simulink model "energy_storage"  (R2018a)
settings: Solver=ode4  StartTime=0.0  StopTime=simu.tTotal  FixedStep=simu.tStep  RelTol=1e-3
undefined symbols (not defined in the file or in its folder): D11, Delta, DiscIntNeverNeededParam, es1, es2, ess, flex, grid, gsc, gt1, ld, sim, simu, u0, Vbase, vsc, WT
libraries: powerlib x40, pwrsys x37, simulink x2, powerlib_meascontrol x2, simulink_extras x1, sps_avr x1
(part 1 of 2)
settings Model: SimulationMode=accelerator  Creator=ericfa  LastModifiedBy=ericfa
settings OptimizationCC: DefaultUnderspecifiedDataType=single
settings DebuggingCC: UnconnectedInputMsg=none  UnconnectedOutputMsg=none  UnconnectedLineMsg=none  UniqueDataStoreMsg=error  StrictBusMsg=ErrorOnBusTreatedAsVector

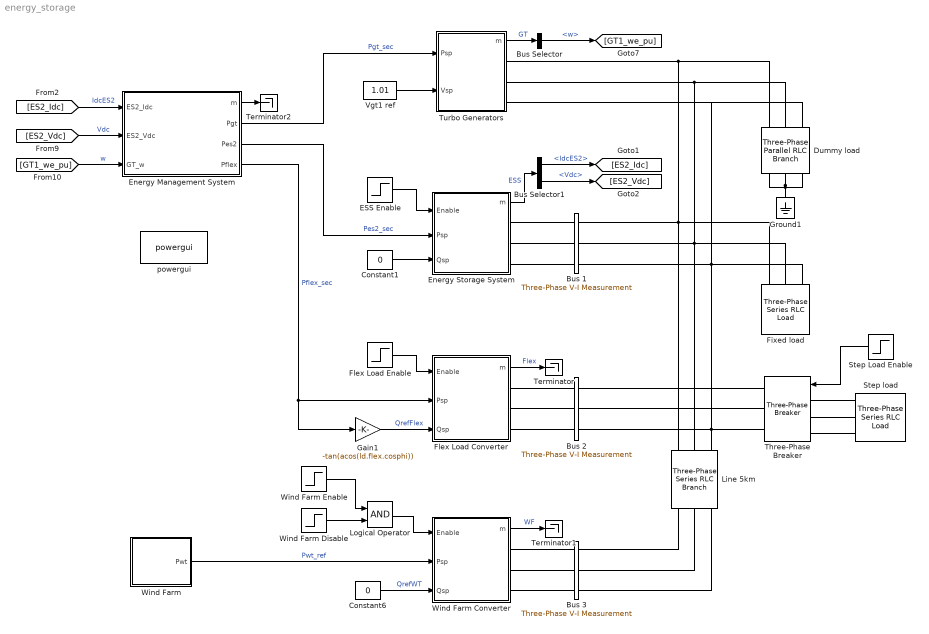
== system energy_storage ==
  Bus Selector : BusSelector  OutputSignals=w
  Bus Selector1 : BusSelector  OutputSignals=IdcES2,Vdc
  Bus 1 : powerlib/Measurements/Three-Phase V-I Measurement  VoltageMeasurement=no  SetLabelV=on  LabelV=Vabc_B2  Vpu=off  VpuLL=off  CurrentMeasurement=no  SetLabelI=on  LabelI=Iabc_B2  Ipu=off  Pbase=100e6  Vbase=500e3  OutputType=Magnitude  PhasorSimulation=off  PSBequivalent=0
      settings: SourceProductName=Simscape Electrical
  Bus 2 : powerlib/Measurements/Three-Phase V-I Measurement  VoltageMeasurement=no  SetLabelV=on  LabelV=Vabc_B2  Vpu=off  VpuLL=off  CurrentMeasurement=no  SetLabelI=on  LabelI=Iabc_B2  Ipu=off  Pbase=100e6  Vbase=500e3  OutputType=Magnitude  PhasorSimulation=off  PSBequivalent=0
      settings: SourceProductName=Simscape Electrical
  Bus 3 : powerlib/Measurements/Three-Phase V-I Measurement  VoltageMeasurement=no  SetLabelV=on  LabelV=Vabc_B2  Vpu=off  VpuLL=off  CurrentMeasurement=no  SetLabelI=on  LabelI=Iabc_B2  Ipu=off  Pbase=100e6  Vbase=500e3  OutputType=Magnitude  PhasorSimulation=off  PSBequivalent=0
      settings: SourceProductName=Simscape Electrical
  Constant1 : Constant  Value=0
  Constant6 : Constant  Value=0
  Dummy load : powerlib/Elements/Three-Phase Parallel RLC Branch  LConnTagsString=A|B|C  RConnTagsString=A|B|C  BranchType=R  Resistance=100*grid.UB2^2/grid.Sb  Inductance=1e-3  Capacitance=1e-6  Measurements=None
      settings: SourceProductName=Simscape Power Systems  SourceProductBaseCode=PS
  ESS Enable : Step  Time=4/grid.fn  SampleTime=0
  Energy Management System : Subsystem
  Energy Storage System : Subsystem
  Fixed load : powerlib/Elements/Three-Phase Series RLC Load  LConnTagsString=A|B|C  Configuration=Delta  NominalVoltage=grid.UB2  Vabc=[1e3 1e3 1e3]  Vabcp=[1e3 1e3 1e3]  NominalFrequency=grid.fn  UnbalancedPower=off  ActivePower=ld.fix.P  InductivePower=tan(acos(ld.fix.cosphi))*ld.fix.P  CapacitivePower=0  Pabc=[10e3 9e3 11e3]  QLabc=[100 90 110]  QCabc=[100 90 110]  Pabcp=[10e3 9e3 11e3]  QLabcp=[100 90 110]  QCabcp=[100 90 110]  Measurements=None  LoadType=constant Z
  Flex Load Converter : Subsystem
  Flex Load Enable : Step  Time=4/grid.fn  SampleTime=0
  Gain1 : Gain  Gain=-tan(acos(ld.flex.cosphi))
  Ground1 : powerlib/Elements/Ground  LConnTagsString=a
  Line 5km : powerlib/Elements/Three-Phase Series RLC Branch  LConnTagsString=A|B|C  RConnTagsString=A|B|C  BranchType=RL  Resistance=0.01273*5  Inductance=5*(0.2337e-3)  Capacitance=1e-6  Measurements=None
  Logical Operator : Logic  AllPortsSameDT=off  OutDataTypeStr=boolean
  Step Load Enable : Step  Time=simu.tLDstep  Before=ld.step.st  After=(1 - ld.step.st)  SampleTime=0
  Step load : powerlib/Elements/Three-Phase Series RLC Load  LConnTagsString=A|B|C  Configuration=Delta  NominalVoltage=grid.UB2  Vabc=[1e3 1e3 1e3]  Vabcp=[1e3 1e3 1e3]  NominalFrequency=grid.fn  UnbalancedPower=off  ActivePower=ld.step.P  InductivePower=tan(acos(ld.fix.cosphi))*ld.step.P  CapacitivePower=0  Pabc=[10e3 9e3 11e3]  QLabc=[100 90 110]  QCabc=[100 90 110]  Pabcp=[10e3 9e3 11e3]  QLabcp=[100 90 110]  QCabcp=[100 90 110]  Measurements=None  LoadType=constant Z
  Terminator : Terminator
  Terminator1 : Terminator
  Terminator2 : Terminator
  Three-Phase Breaker : powerlib/Elements/Three-Phase Breaker  InitialState=open  SwitchA=on  SwitchB=on  SwitchC=on  SwitchTimes="[1/60  5/60]"  External=on  BreakerResistance=0.01  SnubberResistance=1e6  SnubberCapacitance=inf  Measurements=None
  Turbo Generators : Subsystem  SystemSampleTime=10*sim.tStep  mask(Synchronous Generator with Exciter and Governor){SMVn=grid.UB2, SMPn=gt1.SM.Sn, SMcosphi=gt1.SM.cosphi, SMfn=grid.fn, SMp=gt1.SM.p, SMM=gt1.SM.M/2, SMXd=gt1.SM.Xd, SMXdp=gt1.SM.Xdp, SMXdpp=gt1.SM.Xdpp, SMXq=gt1.SM.Xq, SMXqpp=gt1.SM.Xqpp, SMXl=gt1.SM.Xl, SMRs=gt1.SM.Rs, SMTdpSC=gt1.SM.TdpSC, SMTdppSC=gt1.SM.TdppSC, SMTqppSC=gt1.SM.TqppSC, TurbT=gt1.Turb.T, GovKp=gt1.P.Kp, GovKd=gt1.P.Kd, GovTr=gt1.P.Tr, GovFlp=gt1.P.flp, GovDB=gt1.P.DB, ExcTr=gt1.exc.Tr, ExcKa=gt1.exc.Ka, ExcVRMax=gt1.exc.VRmax, ExcVRMin=gt1.exc.VRmin, ExcKf=gt1.exc.Kf, ExcTf=gt1.exc.Tf, ExcTb=gt1.exc.Tb, ExcTc=gt1.exc.Tc, ExcTb1=gt1.exc.Tb1, ExcTc1=gt1.exc.Tc1}
      mask prompts: SMVn "Voltage [V]"; SMPn "Apparent power [VA]"; SMcosphi "Power factor"; SMfn "Frequency [Hz]"; SMp "Pairs of poles"; SMM "Inertia constant [s]"; SMXd "d-axis steady-state"; SMXdp "d-axis transient"; SMXdpp "d-axis subtransient"; SMXq "q-axis steady-state"; SMXqpp "q-axis subtransient"; SMXl "Leakage"; SMRs "Stator (armature) resistance"; SMTdpSC "d-axis transient time"; SMTdppSC "d-axis subtransient time"; SMTqppSC "q-axis subtransient time"; TurbT "Equivalent first-order delay [s]"; GovKp "Permanent droop (primary control)"; GovKd "Transient droop (primary control)"; GovTr "Reset time transient droop (primary control)"; GovFlp "Low-pass frequency [Hz]"; GovDB "Deadband [pu]"; ExcTr "Input filter time constant [s]"; ExcKa "Proportional gain"; ExcVRMax "Maximum output [pu]"; ExcVRMin "Minimum output [pu]"; ExcKf "Rate feedback (derivative) gain"; ExcTf "Rate feedback (reset) time [s]"; ExcTb "1st lag time constant [s]"; ExcTc "1st lead time constant [s]"; ExcTb1 "2nd lag time constant [s]"; ExcTc1 "2nd lead time constant [s]"
      mask DialogControl ParameterGroupVar Prompt: Synchronous Machine
      mask DialogControl Container11_copy Prompt: Rated values
      mask DialogControl Container11 Prompt: Impedances [pu]
      mask DialogControl Container19 Prompt: Short-circuit time constants [s]
      mask DialogControl Container3 Prompt: Turbine
      mask DialogControl Container4 Prompt: Controllers
      mask DialogControl Container6 Prompt: Governor
      mask DialogControl Container8 Prompt: Exciter
  Vgt1 ref : Constant  Value=1.01
  Wind Farm : Subsystem
  Wind Farm Converter : Subsystem
  Wind Farm Disable : Step  Time=simu.tWToff  Before=1  After=0  SampleTime=0
  Wind Farm Enable : Step  Time=4/grid.fn  SampleTime=0
  powergui : powerlib/powergui  Priority=1  SimulationMode=Discrete  SampleTime=simu.tStep  frequency=60  Iterations=50  frequencyindice=0  Pbase=100e6  ErrMax=0.0001  UnitsV=kV  UnitsW=MW  buscounter=0  FunctionMessages=off  echomessages=off  EnableUseOfTLC=off  CurrentSourceSwitches=off  DisableSnubberDevices=off  DisableRonSwitches=off  DisableVfSwitches=off  DisplayEquations=off  SolverType=Tustin/Backward Euler (TBE)  Interpol=off  ExternalGateDelay=off  methode=off  Ts=100  x0status=blocks  SPID=on  SwTol=0  HookPort=off  RestoreLinks=warning  ResistiveCurrentMeasurement=off  Frange=[0:2:500]  Ylog=off  Xlog=on  ShowGrid=off  save=off  variable=ZData  structure=0  ZoomFFT=off  StartTime=0.0  cycles=1  DisplayStyle=1  fundamental=60  FreqAxis=off  MaxFrequency=1000  frequencyindicesteady=1  RmsSteady=2  display=off
  wires:
  ESS Enable/1 -> Energy Storage System/1(Enable)
  Constant1/1 -> Energy Storage System/3(Qsp)
  Vgt1 ref/1 -> Turbo Generators/2(Vsp)
  Gain1/1 -> Flex Load Converter/3(Qsp)  "QrefFlex"
  Flex Load Enable/1 -> Flex Load Converter/1(Enable)
  Energy Management System/4(Pflex) -> Gain1/1, Flex Load Converter/2(Psp)  "Pflex_sec"
  Constant6/1 -> Wind Farm Converter/3(Qsp)  "QrefWT"
  Wind Farm Enable/1 -> Logical Operator/1
  Wind Farm/1(Pwt) -> Wind Farm Converter/2(Psp)  "Pwt_ref"
  Step Load Enable/1 -> Three-Phase Breaker/1
  Bus Selector/1 -> [GT1_we_pu]  "<w>"
  Turbo Generators/1(m) -> Bus Selector/1  "GT"
  Flex Load Converter/1(m) -> Terminator/1  "Flex"
  Wind Farm Converter/1(m) -> Terminator1/1  "WF"
  Bus Selector1/1 -> [ES2_Idc]  "<IdcES2>"
  Energy Storage System/1(m) -> Bus Selector1/1  "ESS"
  Bus Selector1/2 -> [ES2_Vdc]  "<Vdc>"
  [ES2_Idc] -> Energy Management System/1(ES2_Idc)  "IdcES2"
  [ES2_Vdc] -> Energy Management System/2(ES2_Vdc)  "Vdc"
  [GT1_we_pu] -> Energy Management System/3(GT_w)  "w"
  Energy Management System/2(Pgt) -> Turbo Generators/1(Psp)  "Pgt_sec"
  Energy Management System/3(Pes2) -> Energy Storage System/2(Psp)  "Pes2_sec"
  Energy Management System/1(m) -> Terminator2/1
  Wind Farm Disable/1 -> Logical Operator/2
  Logical Operator/1 -> Wind Farm Converter/1(Enable)
  connections:
  Dummy load/LConn2 -- Turbo Generators/RConn2 -- Fixed load/LConn2 -- Three-Phase Breaker/RConn2 -- Line 5km/LConn2 -- Bus 2/RConn2 -- Bus 1/RConn2
  Three-Phase Breaker/RConn3 -- Dummy load/LConn3 -- Turbo Generators/RConn3 -- Fixed load/LConn3 -- Bus 1/RConn3 -- Line 5km/LConn3 -- Bus 2/RConn3
  Energy Storage System/RConn1 -- Bus 1/LConn1
  Energy Storage System/RConn2 -- Bus 1/LConn2
  Energy Storage System/RConn3 -- Bus 1/LConn3
  Dummy load/LConn1 -- Turbo Generators/RConn1 -- Fixed load/LConn1 -- Three-Phase Breaker/RConn1 -- Line 5km/LConn1 -- Bus 2/RConn1 -- Bus 1/RConn1
  Dummy load/RConn2 -- Dummy load/RConn3 -- Dummy load/RConn1 -- Ground1/LConn1
  Flex Load Converter/RConn1 -- Bus 2/LConn1
  Flex Load Converter/RConn2 -- Bus 2/LConn2
  Flex Load Converter/RConn3 -- Bus 2/LConn3
  Wind Farm Converter/RConn3 -- Bus 3/LConn3
  Wind Farm Converter/RConn2 -- Bus 3/LConn2
  Wind Farm Converter/RConn1 -- Bus 3/LConn1
  Bus 3/RConn1 -- Line 5km/RConn1
  Bus 3/RConn2 -- Line 5km/RConn2
  Bus 3/RConn3 -- Line 5km/RConn3
  Step load/LConn1 -- Three-Phase Breaker/LConn1
  Step load/LConn2 -- Three-Phase Breaker/LConn2
  Step load/LConn3 -- Three-Phase Breaker/LConn3

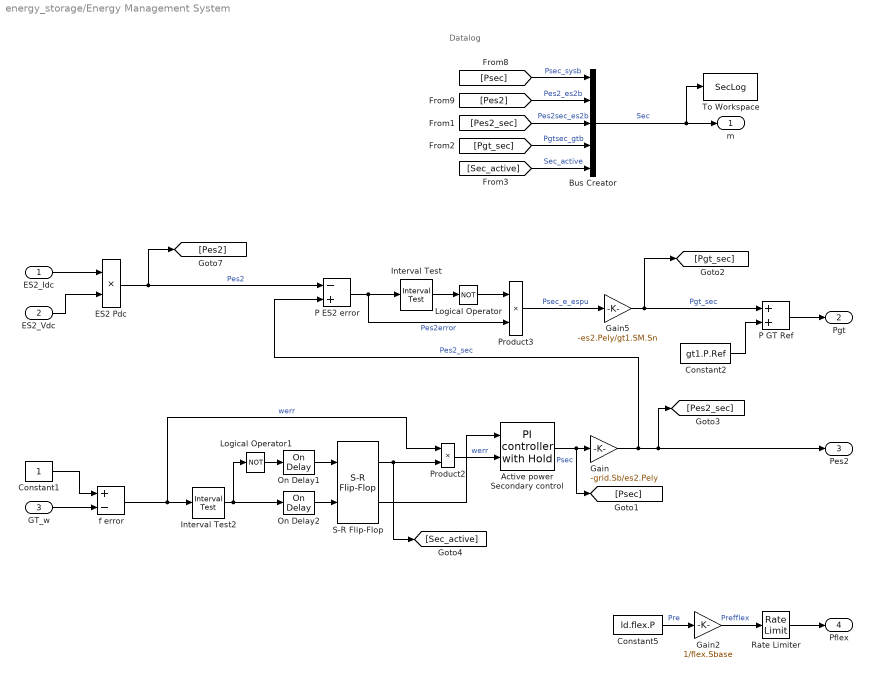
== system energy_storage/Energy Management System ==
  note: Datalog
  ES2_Idc : Inport
  ES2_Vdc : Inport  Port=2
  GT_w : Inport  Port=3
  Active power Secondary control : pwrsys/Controllers/PI controller  with Hold  Kp=0.05  Ki=gt1.P.Ki  Max=(es2.Pfc + gt1.SM.Sn*gt1.SM.cosphi-gt1.P.Ref*gt1.SM.Sn)/grid.Sb  Min=-(es2.Pely+gt1.P.Ref*gt1.SM.Sn)/grid.Sb  x0=0  Ts=10/grid.fn
      settings: SourceProductName=NTNU Power Systems
  Bus Creator : BusCreator  Inputs=5
  Constant1 : Constant
  Constant2 : Constant  Value=gt1.P.Ref
  Constant5 : Constant  Value=ld.flex.P
  ES2 Pdc : Product
  Gain : Gain  Gain=-grid.Sb/es2.Pely
  Gain2 : Gain  Gain=1/flex.Sbase
  Gain5 : Gain  Gain=-es2.Pely/gt1.SM.Sn
  Interval Test : simulink/Logic and Bit Operations/Interval Test  IntervalClosedRight=on  uplimit=0.05  IntervalClosedLeft=on  lowlimit=-0.05  OutDataTypeStr=boolean
  Interval Test2 : simulink/Logic and Bit Operations/Interval Test  IntervalClosedRight=on  uplimit=0.005  IntervalClosedLeft=on  lowlimit=-0.005  OutDataTypeStr=boolean
  Logical Operator : Logic  Operator=NOT  AllPortsSameDT=off  OutDataTypeStr=boolean
  Logical Operator1 : Logic  Operator=NOT  AllPortsSameDT=off  OutDataTypeStr=boolean
  On Delay1 : powerlib_meascontrol/Logic/On Delay  DelayType=On delay  delay=30  ic=0  Ts=10/grid.fn
      settings: SourceProductName=Simscape Power Systems
  On Delay2 : powerlib_meascontrol/Logic/On Delay  DelayType=On delay  delay=60  ic=0  Ts=10/grid.fn
      settings: SourceProductName=Simscape Power Systems
  P ES2 error : Sum  Inputs=-+
  P GT Ref : Sum
  Product2 : Product
  Product3 : Product
  Rate Limiter : RateLimiter  RisingSlewLimit=100  FallingSlewLimit=-100  SampleTimeMode=inherited
  S-R Flip-Flop : simulink_extras/Flip Flops/S-R Flip-Flop  initial_condition=0
  To Workspace : ToWorkspace  VariableName=SecLog  SaveFormat=Timeseries  SampleTime=-1
      settings: Decimation=2000
  f error : Sum  Inputs=+-
  m : Outport
  Pgt : Outport  Port=2
  Pes2 : Outport  Port=3
  Pflex : Outport  Port=4
  wires:
  Constant1/1 -> f error/1
  Product2/1 -> Active power Secondary control/2  "werr"
  Product3/1 -> Gain5/1  "Psec_e_espu"
  Gain/1 -> [Pes2_sec], Pes2/1, P ES2 error/2  "Pes2_sec"
  P ES2 error/1 -> Interval Test/1, Product3/2  "Pes2error"
  Active power Secondary control/1 -> [Psec], Gain/1  "Psec"
  Interval Test2/1 -> Logical Operator1/1, On Delay2/1
  S-R Flip-Flop/2 -> Active power Secondary control/1
  GT_w/1 -> f error/2
  On Delay2/1 -> S-R Flip-Flop/2
  Logical Operator1/1 -> On Delay1/1
  f error/1 -> Product2/1, Interval Test2/1  "werr"
  S-R Flip-Flop/1 -> [Sec_active], Product2/2
  Interval Test/1 -> Logical Operator/1
  Logical Operator/1 -> Product3/1
  On Delay1/1 -> S-R Flip-Flop/1
  ES2 Pdc/1 -> [Pes2], P ES2 error/1  "Pes2"
  ES2_Idc/1 -> ES2 Pdc/1
  ES2_Vdc/1 -> ES2 Pdc/2
  Gain5/1 -> P GT Ref/1, [Pgt_sec]  "Pgt_sec"
  Bus Creator/1 -> To Workspace/1, m/1  "Sec"
  [Pes2_sec] -> Bus Creator/3  "Pes2sec_es2b"
  [Pgt_sec] -> Bus Creator/4  "Pgtsec_gtb"
  [Psec] -> Bus Creator/1  "Psec_sysb"
  [Pes2] -> Bus Creator/2  "Pes2_es2b"
  [Sec_active] -> Bus Creator/5  "Sec_active"
  Constant5/1 -> Gain2/1  "Pre"
  Gain2/1 -> Rate Limiter/1  "Prefflex"
  Rate Limiter/1 -> Pflex/1
  Constant2/1 -> P GT Ref/2
  P GT Ref/1 -> Pgt/1

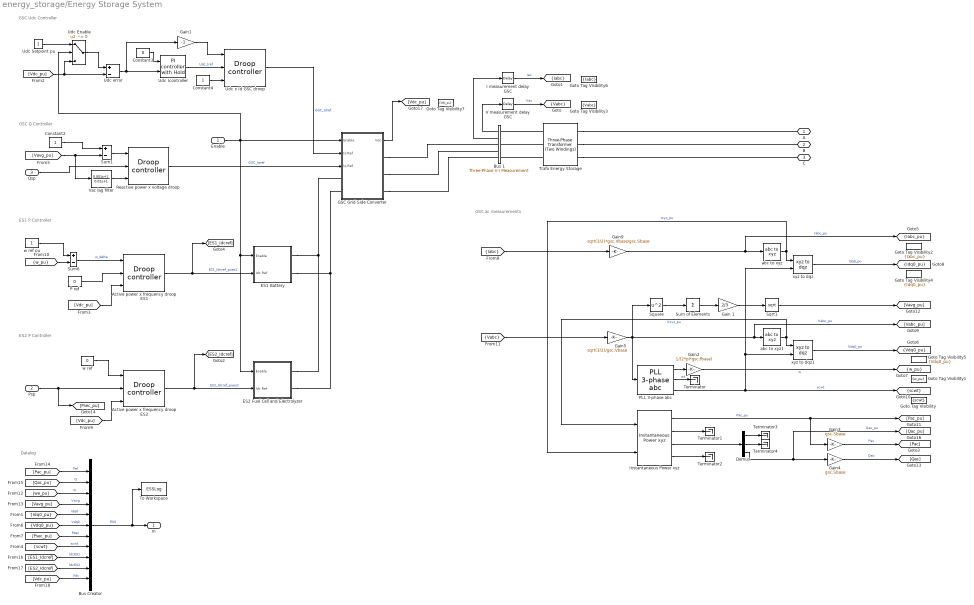
== system energy_storage/Energy Storage System ==
  note: GSC ac measurements
  note: ES1 P Controller
  note: GSC Q Controller
  note: GSC Udc Controller
  note: ES2 P Controller
  note: Datalog
  Enable : Inport
  Psp : Inport  Port=2
  Qsp : Inport  Port=3
  Active power x frequency droop ES1 : pwrsys/Controllers/Droop controller  Refmax=1  Refmin=-1  Ts=-1  Kp=ess.P.Kp  Kd=0  Tr=ess.P.Tr  flp=ess.P.flp  DB=ess.P.DB
      settings: SourceProductName=NTNU Power Systems
  Active power x frequency droop ES2 : pwrsys/Controllers/Droop controller  Refmax=1  Refmin=-es2.Pfc/es2.Pely  Ts=-1  Kp=0  Kd=0  Tr=ess.P.Tr  flp=ess.P.flp  DB=ess.P.DB
      settings: SourceProductName=NTNU Power Systems
  Bus Creator : BusCreator  Inputs=11
  Bus 1 : powerlib/Measurements/Three-Phase V-I Measurement  VoltageMeasurement=phase-to-ground  SetLabelV=off  LabelV=Vabc  Vpu=off  VpuLL=off  CurrentMeasurement=yes  SetLabelI=off  LabelI=Iabc  Ipu=off  Pbase=Sbase  Vbase=Vbase*sqrt(3/2)  OutputType=Complex  PhasorSimulation=off  PSBequivalent=0
  Constant2 : Constant
  Constant3 : Constant  Value=0
  Constant4 : Constant
  Demux : Demux  Outputs=3
  ES1 Battery : Subsystem
  ES2 Fuel Cell and Electrolyzer : Subsystem
  GSC Grid Side Converter : Subsystem
  "Gain 1 " : Gain  Gain=2/3
  Gain1 : Gain  Gain=-1
  Gain2 : Gain  Gain=1/(2*pi*gsc.fbase)
  Gain3 : Gain  Gain=gsc.Sbase
  Gain4 : Gain  Gain=gsc.Sbase
  Gain5 : Gain  Gain=sqrt(3/2)/gsc.Vbase
  Gain9 : Gain  Gain=sqrt(3/2)*gsc.Vbase/gsc.Sbase
  Goto Tag Visibility : GotoTagVisibility  GotoTag=scwt
  Goto Tag Visibility1 : GotoTagVisibility  GotoTag=w_pu
  Goto Tag Visibility2 : GotoTagVisibility  GotoTag=Iabc_pu
  Goto Tag Visibility3 : GotoTagVisibility  GotoTag=Vabc
  Goto Tag Visibility4 : GotoTagVisibility  GotoTag=Idq0_pu
  Goto Tag Visibility5 : GotoTagVisibility  GotoTag=Vdq0_pu
  Goto Tag Visibility6 : GotoTagVisibility  GotoTag=Iabc
  Goto Tag Visibility7 : GotoTagVisibility  GotoTag=Vdc_pu
  I measurement delay GSC : TransportDelay  DelayTime=simu.tStep
  Instantaneous Power xyz : pwrsys/Measurement/Instantaneous Power xyz  typeTransf=Amplitude-invariant
      settings: SourceProductName=NTNU Power Systems
  P ref : Constant  Value=0
  PLL 3-phase abc : pwrsys/PLLs/PLL 3-phase abc  fnom=gsc.fbase  fdev=1/3*gsc.fbase  zeta=0.707  Kp=gsc.pll.Kp  Ki=gsc.pll.Ki  Kd=gsc.pll.Kd  Tr=gsc.pll.Tr  Ts=gsc.fSwitch  wt0=0
      settings: SourceProductName=NTNU Power Systems
  Reactive power x voltage droop : pwrsys/Controllers/Droop controller  Refmax=1  Refmin=-1  Ts=-1  Kp=ess.Q.Kp  Kd=ess.Q.Kd  Tr=ess.Q.Tr  flp=ess.Q.flp  DB=ess.Q.DB
      settings: SourceProductName=NTNU Power Systems
  Sqrt1 : Sqrt  SaturateOnIntegerOverflow=on
  Square : Math  Operator=square  SaturateOnIntegerOverflow=on
  Sum of Elements : Sum  Inputs=+
  Sum1 : Sum  Inputs=+-
  Sum6 : Sum  Inputs=+-
  Terminator{,1..4} (5 alike) : Terminator
  To Workspace : ToWorkspace  VariableName=ESSLog  SaveFormat=Timeseries  SampleTime=-1
      settings: Decimation=20
  Trafo Energy Storage : powerlib/Elements/Three-Phase Transformer (Two Windings)  Winding1Connection=Yg  Winding2Connection=Delta (D11)  CoreType=Three single-phase transformers  SetSaturation=off  Hysteresis=off  DataFile='hysteresis'  SetInitialFlux=off  Measurements=None  UNITS=pu  NominalPower=[ gsc.Sbase , grid.fn ]  Winding1=[ grid.UB1 , 0.002 , gsc.filterpu.Lg/2 ]  Winding2=[ grid.UB2 , 0.002 , gsc.filterpu.Lg/2 ]  Rm=200  Lm=200  L0=0.5  Saturation=[ 0,0 ; 0.0024,1.2 ; 1.0,1.52 ]  InitialFluxes=[ 0.8 , -0.8 , 0.7 ]  MoreParameters=off  BreakLoop=off  DataType=off  TransfoNumber=1
  Udc Enable : Switch  Criteria=u2 ~= 0
  Udc Icontroller : pwrsys/Controllers/PI controller  with Hold  Kp=0  Ki=ess.Udc.Ki  Max=1  Min=-1  x0=0  Ts=-1
      settings: SourceProductName=NTNU Power Systems
  Udc Setpoint pu : Constant
  Udc error : Sum  Inputs=+-
  "Udc x Id GSC droop " : pwrsys/Controllers/Droop controller  Refmax=1  Refmin=-1  Ts=-1  Kp=ess.Udc.Kp  Kd=ess.Udc.Kd  Tr=ess.Udc.Tr  flp=ess.Udc.flp  DB=ess.Udc.DB
      settings: SourceProductName=NTNU Power Systems
  V measurement delay GSC : TransportDelay  DelayTime=simu.tStep
  Vac lag filter : TransferFcn  Numerator=[0.001 1]  Denominator=[0.01 1]
  abc to xyz : pwrsys/Transformations/abc to xyz  typeTransf=Amplitude-invariant
      settings: SourceProductName=NTNU Power Systems
  abc to xyz1 : pwrsys/Transformations/abc to xyz  typeTransf=Amplitude-invariant
      settings: SourceProductName=NTNU Power Systems
  "w ref " : Constant  Value=0
  w ref pu : Constant
  xyz to dqz : pwrsys/Transformations/xyz to dqz  SystemSampleTime=-1
      settings: SourceProductName=NTNU Power Systems
  xyz to dqz1 : pwrsys/Transformations/xyz to dqz  SystemSampleTime=-1
      settings: SourceProductName=NTNU Power Systems
  A : PMIOPort  Side=Right
  B : PMIOPort  Port=2  Side=Right
  C : PMIOPort  Port=3  Side=Right
  m : Outport
  tag scope: Iabc=scoped, Iabc_pu=scoped, Idq0_pu=scoped, Vabc=scoped, Vdq0_pu=scoped, scwt=scoped, w_pu=scoped
  wires:
  Constant3/1 -> Udc Icontroller/1
  Udc Enable/1 -> Udc error/1
  Udc Setpoint pu/1 -> Udc Enable/1
  Udc error/1 -> Gain1/1, Udc Icontroller/2
  "Udc x Id GSC droop "/1 -> GSC Grid Side Converter/2(Id Ref)  "GSC_Idref"
  I measurement delay GSC/1 -> [Iabc]  "Iac"
  Active power x frequency droop ES1/1 -> ES1 Battery/2(Idc Ref), [ES1_Idcref]  "ES1_Idcref_pues1"
  [Vdc_pu] -> Udc Enable/3, Udc error/2
  V measurement delay GSC/1 -> [Vabc]  "Vac"
  Bus 1/1 -> V measurement delay GSC/1
  Udc Icontroller/1 -> "Udc x Id GSC droop "/2  "Udc_Iref"
  Constant2/1 -> Sum1/1
  w ref pu/1 -> Sum6/1
  Sum1/1 -> Reactive power x voltage droop/1
  Gain1/1 -> "Udc x Id GSC droop "/1
  Bus 1/2 -> I measurement delay GSC/1
  [w_pu] -> Sum6/2
  Sum6/1 -> Active power x frequency droop ES1/1  "w_delta"
  [Vdc_pu] -> Active power x frequency droop ES1/3
  Enable/1 -> ES2 Fuel Cell and Electrolyzer/1(Enable), ES1 Battery/1(Enable), GSC Grid Side Converter/1(Enable), Udc Enable/2
  Constant4/1 -> "Udc x Id GSC droop "/3
  Reactive power x voltage droop/1 -> GSC Grid Side Converter/3(Iq Ref)  "GSC_Iqref"
  [Vdc_pu] -> Active power x frequency droop ES2/3
  Active power x frequency droop ES2/1 -> ES2 Fuel Cell and Electrolyzer/2(Idc Ref), [ES2_Idcref]  "ES2_Idcref_pues2"
  "w ref "/1 -> Active power x frequency droop ES2/1
  P ref/1 -> Active power x frequency droop ES1/2
  [Vavg_pu] -> Vac lag filter/1, Sum1/2
  Vac lag filter/1 -> Reactive power x voltage droop/3
  Psp/1 -> [Psec_pu], Active power x frequency droop ES2/2
  Qsp/1 -> Reactive power x voltage droop/2
  Sqrt1/1 -> [Vavg_pu]
  Gain9/1 -> [Iabc_pu], abc to xyz/1  "Iabc_pu"
  xyz to dqz/1 -> [Idq0_pu]  "Idq0_pu"
  Gain5/1 -> Square/1, PLL 3-phase abc/1, [Vabc_pu], abc to xyz1/1  "Vabc_pu"
  PLL 3-phase abc/3 -> [scwt], xyz to dqz/2, xyz to dqz1/2  "scwt"
  Gain2/1 -> [w_pu]  "w"
  PLL 3-phase abc/1 -> Gain2/1
  xyz to dqz1/1 -> [Vdq0_pu]  "Vdq0_pu"
  [Iabc] -> Gain9/1
  [Vabc] -> Gain5/1
  Instantaneous Power xyz/1 -> Gain3/1, [Pac_pu]  "Pac_pu"
  Demux/3 -> [Qac_pu], Gain4/1  "Qac_pu"
  Square/1 -> Sum of Elements/1
  Sum of Elements/1 -> "Gain 1 "/1
  "Gain 1 "/1 -> Sqrt1/1
  abc to xyz/1 -> xyz to dqz/1, Instantaneous Power xyz/2  "Ixyz_pu"
  abc to xyz1/1 -> xyz to dqz1/1, Instantaneous Power xyz/1  "Vxyz_pu"
  PLL 3-phase abc/2 -> Terminator/1  "wt"
  Instantaneous Power xyz/2 -> Terminator1/1
  Instantaneous Power xyz/4 -> Terminator2/1
  Instantaneous Power xyz/3 -> Demux/1
  Demux/1 -> Terminator3/1
  Demux/2 -> Terminator4/1
  Gain3/1 -> [Pac]  "Pac"
  Gain4/1 -> [Qac]  "Qac"
  GSC Grid Side Converter/1(Vdc) -> [Vdc_pu]
  Bus Creator/1 -> To Workspace/1, m/1  "ESS"
  [Vavg_pu] -> Bus Creator/4  "Vavg"
  [Pac_pu] -> Bus Creator/1  "Pel"
  [Psec_pu] -> Bus Creator/7  "Psec"
  [Vdq0_pu] -> Bus Creator/6  "Vdq0"
  [Idq0_pu] -> Bus Creator/5  "Idq0"
  [Qac_pu] -> Bus Creator/2  "Q"
  [scwt] -> Bus Creator/8  "scwt"
  [we_pu] -> Bus Creator/3  "w"
  [ES1_Idcref] -> Bus Creator/9  "IdcES1"
  [ES2_Idcref] -> Bus Creator/10  "IdcES2"
  [Vdc_pu] -> Bus Creator/11  "Vdc"
  connections:
  ES1 Battery/RConn2 -- ES2 Fuel Cell and Electrolyzer/RConn2 -- GSC Grid Side Converter/LConn2
  Trafo Energy Storage/LConn2 -- Bus 1/LConn2
  GSC Grid Side Converter/RConn3 -- Bus 1/RConn3
  GSC Grid Side Converter/RConn1 -- Bus 1/RConn1
  Trafo Energy Storage/LConn3 -- Bus 1/LConn3
  GSC Grid Side Converter/RConn2 -- Bus 1/RConn2
  Trafo Energy Storage/LConn1 -- Bus 1/LConn1
  Trafo Energy Storage/RConn3 -- C/RConn1
  Trafo Energy Storage/RConn2 -- B/RConn1
  Trafo Energy Storage/RConn1 -- A/RConn1
  ES1 Battery/RConn1 -- ES2 Fuel Cell and Electrolyzer/RConn1 -- GSC Grid Side Converter/LConn1

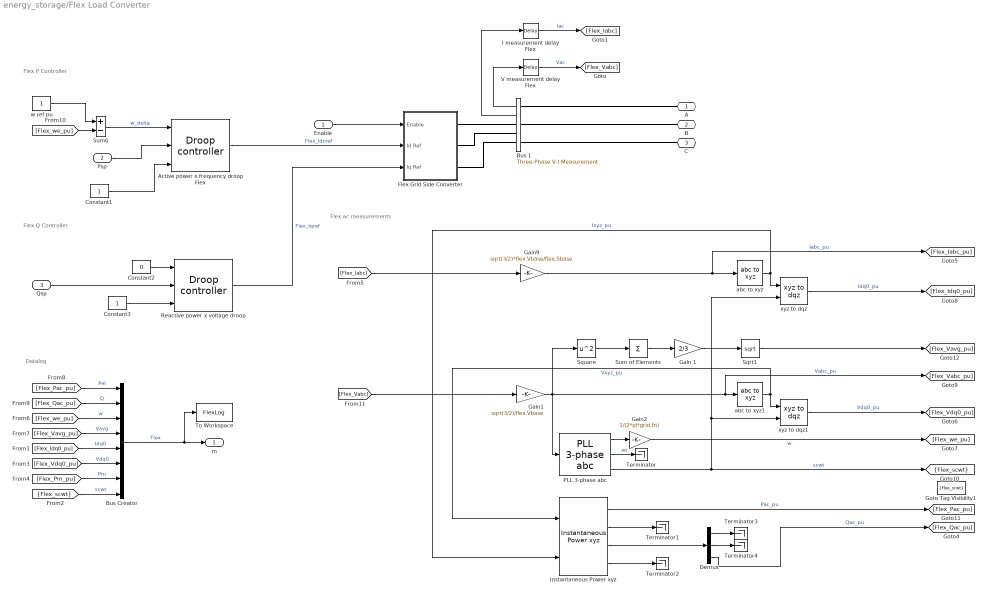
== system energy_storage/Flex Load Converter ==
  note: Flex ac measurements
  note: Flex P Controller
  note: Flex Q Controller
  note: Datalog
  Enable : Inport
  Psp : Inport  Port=2
  Qsp : Inport  Port=3
  Active power x frequency droop Flex : pwrsys/Controllers/Droop controller  Refmax=1  Refmin=0  Ts=-1  Kp=flex.P.Kp  Kd=0  Tr=flex.P.Tr  flp=flex.P.flp  DB=flex.P.DB
      settings: SourceProductName=NTNU Power Systems
  Bus Creator : BusCreator  Inputs=8
  Bus 1 : powerlib/Measurements/Three-Phase V-I Measurement  VoltageMeasurement=phase-to-ground  SetLabelV=off  LabelV=Vabc  Vpu=off  VpuLL=off  CurrentMeasurement=yes  SetLabelI=off  LabelI=Iabc  Ipu=off  Pbase=Sbase  Vbase=Vbase*sqrt(3/2)  OutputType=Complex  PhasorSimulation=off  PSBequivalent=0
  Constant1 : Constant
  Constant2 : Constant  Value=0
  Constant3 : Constant
  Demux : Demux  Outputs=3
  Flex Grid Side Converter : Subsystem
  "Gain 1 " : Gain  Gain=2/3
  Gain1 : Gain  Gain=sqrt(3/2)/flex.Vbase
  Gain2 : Gain  Gain=1/(2*pi*grid.fn)
  Gain9 : Gain  Gain=sqrt(3/2)*flex.Vbase/flex.Sbase
  Goto Tag Visibility1 : GotoTagVisibility  GotoTag=Flex_scwt
  I measurement delay Flex : TransportDelay  DelayTime=simu.tStep
  Instantaneous Power xyz : pwrsys/Measurement/Instantaneous Power xyz  typeTransf=Amplitude-invariant
      settings: SourceProductName=NTNU Power Systems
  PLL 3-phase abc : pwrsys/PLLs/PLL 3-phase abc  fnom=gsc.fbase  fdev=1/3*gsc.fbase  zeta=0.707  Kp=gsc.pll.Kp  Ki=gsc.pll.Ki  Kd=gsc.pll.Kd  Tr=gsc.pll.Tr  Ts=gsc.fSwitch  wt0=0
      settings: SourceProductName=NTNU Power Systems
  Reactive power x voltage droop : pwrsys/Controllers/Droop controller  Refmax=0.5  Refmin=-0.5  Ts=-1  Kp=0  Kd=0  Tr=1  flp=1  DB=0
      settings: SourceProductName=NTNU Power Systems
  Sqrt1 : Sqrt  SaturateOnIntegerOverflow=on
  Square : Math  Operator=square  SaturateOnIntegerOverflow=on
  Sum of Elements : Sum  Inputs=+
  Sum6 : Sum  Inputs=+-
  Terminator{,1..4} (5 alike) : Terminator
  To Workspace : ToWorkspace  VariableName=FlexLog  SaveFormat=Timeseries  SampleTime=-1
      settings: Decimation=20
  V measurement delay Flex : TransportDelay  DelayTime=simu.tStep
  abc to xyz : pwrsys/Transformations/abc to xyz  typeTransf=Amplitude-invariant
      settings: SourceProductName=NTNU Power Systems
  abc to xyz1 : pwrsys/Transformations/abc to xyz  typeTransf=Amplitude-invariant
      settings: SourceProductName=NTNU Power Systems
  w ref pu : Constant
  xyz to dqz : pwrsys/Transformations/xyz to dqz  SystemSampleTime=-1
      settings: SourceProductName=NTNU Power Systems
  xyz to dqz1 : pwrsys/Transformations/xyz to dqz  SystemSampleTime=-1
      settings: SourceProductName=NTNU Power Systems
  A : PMIOPort  Side=Right
  B : PMIOPort  Port=2  Side=Right
  C : PMIOPort  Port=3  Side=Right
  m : Outport
  tag scope: Flex_scwt=scoped
  wires:
  I measurement delay Flex/1 -> [Flex_Iabc]  "Iac"
  Active power x frequency droop Flex/1 -> Flex Grid Side Converter/2(Id Ref)  "Flex_Idcref"
  Enable/1 -> Flex Grid Side Converter/1(Enable)
  V measurement delay Flex/1 -> [Flex_Vabc]  "Vac"
  Bus 1/1 -> V measurement delay Flex/1
  Constant3/1 -> Reactive power x voltage droop/3
  w ref pu/1 -> Sum6/1
  Constant2/1 -> Reactive power x voltage droop/1
  Qsp/1 -> Reactive power x voltage droop/2
  Bus 1/2 -> I measurement delay Flex/1
  [Flex_we_pu] -> Sum6/2
  Sum6/1 -> Active power x frequency droop Flex/1  "w_delta"
  Constant1/1 -> Active power x frequency droop Flex/3
  Reactive power x voltage droop/1 -> Flex Grid Side Converter/3(Iq Ref)  "Flex_Iqref"
  Psp/1 -> Active power x frequency droop Flex/2
  [Flex_scwt] -> Bus Creator/8  "scwt"
  [Flex_we_pu] -> Bus Creator/3  "w"
  [Flex_Vdq0_pu] -> Bus Creator/6  "Vdq0"
  [Flex_Idq0_pu] -> Bus Creator/5  "Idq0"
  [Flex_Qac_pu] -> Bus Creator/2  "Q"
  [Flex_Pm_pu] -> Bus Creator/7  "Pm"
  [Flex_Vavg_pu] -> Bus Creator/4  "Vavg"
  Bus Creator/1 -> To Workspace/1, m/1  "Flex"
  [Flex_Pac_pu] -> Bus Creator/1  "Pel"
  Sqrt1/1 -> [Flex_Vavg_pu]
  Gain9/1 -> [Flex_Iabc_pu], abc to xyz/1  "Iabc_pu"
  xyz to dqz/1 -> [Flex_Idq0_pu]  "Idq0_pu"
  Gain1/1 -> Square/1, PLL 3-phase abc/1, [Flex_Vabc_pu], abc to xyz1/1  "Vabc_pu"
  PLL 3-phase abc/3 -> [Flex_scwt], xyz to dqz/2, xyz to dqz1/2  "scwt"
  Gain2/1 -> [Flex_we_pu]  "w"
  PLL 3-phase abc/1 -> Gain2/1
  xyz to dqz1/1 -> [Flex_Vdq0_pu]  "Vdq0_pu"
  [Flex_Iabc] -> Gain9/1
  [Flex_Vabc] -> Gain1/1
  Instantaneous Power xyz/1 -> [Flex_Pac_pu]  "Pac_pu"
  Demux/3 -> [Flex_Qac_pu]  "Qac_pu"
  Square/1 -> Sum of Elements/1
  Sum of Elements/1 -> "Gain 1 "/1
  "Gain 1 "/1 -> Sqrt1/1
  abc to xyz/1 -> xyz to dqz/1, Instantaneous Power xyz/2  "Ixyz_pu"
  abc to xyz1/1 -> xyz to dqz1/1, Instantaneous Power xyz/1  "Vxyz_pu"
  PLL 3-phase abc/2 -> Terminator/1  "wt"
  Instantaneous Power xyz/2 -> Terminator1/1
  Instantaneous Power xyz/4 -> Terminator2/1
  Instantaneous Power xyz/3 -> Demux/1
  Demux/1 -> Terminator3/1
  Demux/2 -> Terminator4/1
  connections:
  B/RConn1 -- Bus 1/LConn2
  Bus 1/RConn3 -- Flex Grid Side Converter/RConn3
  Bus 1/RConn1 -- Flex Grid Side Converter/RConn1
  C/RConn1 -- Bus 1/LConn3
  Bus 1/RConn2 -- Flex Grid Side Converter/RConn2
  A/RConn1 -- Bus 1/LConn1

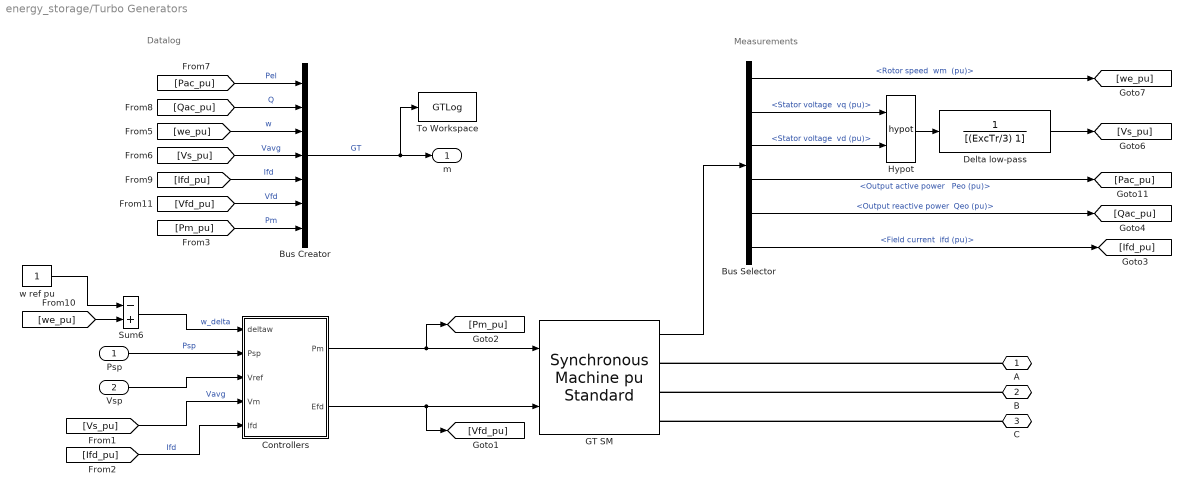
== system energy_storage/Turbo Generators ==
  note: Measurements
  note: Datalog
  Psp : Inport
  Vsp : Inport  Port=2
  Bus Creator : BusCreator  Inputs=7
  Bus Selector : BusSelector  OutputSignals="Mechanical.Rotor speed  wm  (pu),dq0 components.Stator voltage  vq (pu),dq0 components.Stator voltage  vd (pu),Output active power   Peo (pu),Output reactive power  Qeo (pu),dq0 components.Field current  ifd (pu)"
  Controllers : Subsystem  SystemSampleTime=1/(20*grid.fn)
  Delta low-pass : TransferFcn  Denominator=[(ExcTr/3) 1]
  GT SM : powerlib/Machines/Synchronous Machine pu Standard  PresetModel=No  MechanicalLoad=Mechanical power Pm  ShowDetailedParameters=on  RotorType=Salient-pole  Units=per unit standard parameters  MeasurementBus=off  NominalParameters=[SMPn SMVn SMfn]  Reactances1=[ 2.12, 0.299, 0.188, 1.76, 0.65, 0.25, 0.15 ]  Reactances2=[SMXd SMXdp SMXdpp SMXq SMXqpp SMXl]  dAxisTimeConstants=Short-circuit  qAxisTimeConstants=Short-circuit  TimeConstants1="[ 4.4849  0.0681  0.1  ]"  TimeConstants2=[ 8.0, 0.03, 1.0, 0.07 ]  TimeConstants3="[  4.49  0.0681  0.0513  ]"  TimeConstants4=[ 8.0, 0.03, 0.3371, 0.0295 ]  TimeConstants5=[ 1.01, 0.053, 0.1 ]  TimeConstants6=[ 1.3201, 0.023, 1.0, 0.07 ]  TimeConstants7=[SMTdpSC SMTdppSC SMTqppSC]  TimeConstants8=[ 1.3201, 0.0231, 0.3371, 0.0295 ]  StatorResistance=SMRs  Mechanical=[SMM 0 SMp]  PolePairs=20  InitialConditions=[0 -67.7688 0.420455 0.420455 0.420455 0 -120 120 sqrt(3/2)*1.27233]  SetSaturation=on  Saturation=[0.6404,0.7127,0.8441,0.9214,0.9956,1.082,1.19,1.316,1.457;0.7,0.7698,0.8872,0.9466,0.9969,1.046,1.1,1.151,1.201]  LoadFlowParameters=[2 37000000 0 0 0]  TsPowergui=0  TsBlock=-1  IterativeModel=Trapezoidal non iterative  IterativeDiscreteModel=Trapezoidal non iterative  BusType=swing  Pref=0  Qref=0  Qmin=-inf  Qmax=inf  PLF=0  QLF=0
      settings: SourceProductName=Simscape Power Systems
  Hypot : Math  Operator=hypot  SaturateOnIntegerOverflow=on
  Sum6 : Sum  Inputs=-+
  To Workspace : ToWorkspace  VariableName=GTLog  SaveFormat=Timeseries  SampleTime=-1
      settings: Decimation=20
  w ref pu : Constant
  A : PMIOPort  Side=Right
  B : PMIOPort  Port=2  Side=Right
  C : PMIOPort  Port=3  Side=Right
  m : Outport
  wires:
  [we_pu] -> Sum6/2
  w ref pu/1 -> Sum6/1
  Delta low-pass/1 -> [Vs_pu]
  Bus Selector/6 -> [Ifd_pu]  "<Field current  ifd (pu)>"
  GT SM/1 -> Bus Selector/1
  Bus Selector/5 -> [Qac_pu]  "<Output reactive power  Qeo (pu)>"
  Bus Selector/3 -> Hypot/2  "<Stator voltage  vd (pu)>"
  Bus Selector/2 -> Hypot/1  "<Stator voltage  vq (pu)>"
  Bus Selector/1 -> [we_pu]  "<Rotor speed  wm  (pu)>"
  Hypot/1 -> Delta low-pass/1
  Bus Selector/4 -> [Pac_pu]  "<Output active power   Peo (pu)>"
  [Vs_pu] -> Bus Creator/4  "Vavg"
  [Pac_pu] -> Bus Creator/1  "Pel"
  [Qac_pu] -> Bus Creator/2  "Q"
  [we_pu] -> Bus Creator/3  "w"
  [Ifd_pu] -> Bus Creator/5  "Ifd"
  [Vfd_pu] -> Bus Creator/6  "Vfd"
  Bus Creator/1 -> To Workspace/1, m/1  "GT"
  Sum6/1 -> Controllers/1(deltaw)  "w_delta"
  Psp/1 -> Controllers/2(Psp)  "Psp"
  Vsp/1 -> Controllers/3(Vref)
  [Vs_pu] -> Controllers/4(Vm)  "Vavg"
  [Ifd_pu] -> Controllers/5(Ifd)  "Ifd"
  [Pm_pu] -> Bus Creator/7  "Pm"
  Controllers/1(Pm) -> [Pm_pu], GT SM/1
  Controllers/2(Efd) -> [Vfd_pu], GT SM/2
  connections:
  B/RConn1 -- GT SM/RConn2
  A/RConn1 -- GT SM/RConn1
  C/RConn1 -- GT SM/RConn3

== system energy_storage/Wind Farm ==
  note: Wind Turbine
  Add : Sum  Inputs=-+
  First order delay : DiscreteIntegrator  gainval=1  InitialCondition=WT.wspeed  SampleTime=-1  ICPrevOutput=DiscIntNeverNeededParam  ICPrevScaledInput=DiscIntNeverNeededParam
  Gain4 : Gain  Gain=-WT.Prated/WT.Sbase
  Inertia : Constant  Value=WT.Tlp
  Power curve pu : Lookup  InputValues=WT.pcurve.wind  Table=WT.pcurve.power
  Product : Product  Inputs=*/
  Product1 : Product  Inputs=/*
  Rate Limiter1 : RateLimiter  RisingSlewLimit=100  FallingSlewLimit=-100  SampleTimeMode=inherited
  Wind Model Kaimal spectrum according to IEC61400-1 : Subsystem  TreatAsAtomicUnit=on  mask(Wind Model using Simulink Band-limited white noise generator){D_rotor=WT.Rdiam, L=WT.Lmm, turb_int=WT.Turb, T_sample=1/grid.fn}
      mask prompts: D_rotor "Rotor diameter [m]"; L "Length scale [m]"; turb_int "Turbulence intensity [%]"; T_sample "Sample time [sec]"
      mask help:
      | Implements a rotor wind model developped by RISOE National Laboratory based on Kaimal spectra. The model takes into account the rotational turbulences and the tower shadow.
      | This model uses the built-in band-limited white noise generator from Simulink
      mask init:
      | r = D_rotor/2;
      mask Display: disp('Wind\nModel')
  Wind Speed : Constant  Value=WT.wspeed
  Pwt : Outport
  wires:
  Product/1 -> First order delay/1
  Add/1 -> Product/1
  Wind Model Kaimal spectrum according to IEC61400-1/1(wind) -> Product1/1, Add/2
  Inertia/1 -> Product1/2
  Product1/1 -> Product/2
  First order delay/1 -> Power curve pu/1, Add/1
  Wind Speed/1 -> Wind Model Kaimal spectrum according to IEC61400-1/1(avg_wind)
  Gain4/1 -> Rate Limiter1/1  "PrefWT"
  Power curve pu/1 -> Gain4/1  "Pre"
  Rate Limiter1/1 -> Pwt/1

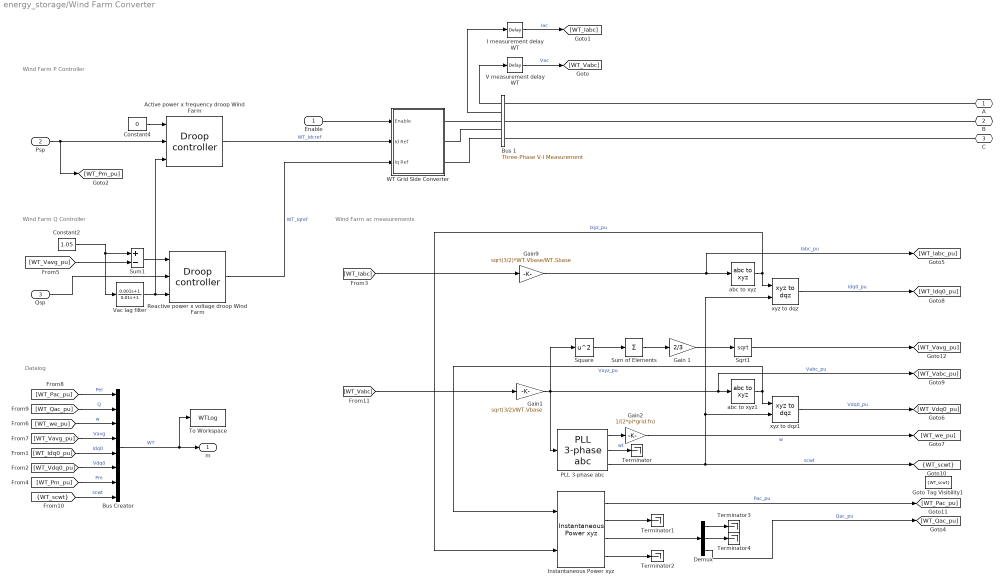
== system energy_storage/Wind Farm Converter ==
  note: Wind Farm ac
      | measurements
  note: Wind Farm P Controller
  note: Wind Farm Q Controller
  note: Datalog
  Enable : Inport
  Psp : Inport  Port=2
  Qsp : Inport  Port=3
  Active power x frequency droop Wind Farm : pwrsys/Controllers/Droop controller  Refmax=0  Refmin=-WT.cosphi  Ts=-1  Kp=0  Kd=0  Tr=100  flp=1  DB=0
      settings: SourceProductName=NTNU Power Systems
  Bus Creator : BusCreator  Inputs=8
  Bus 1 : powerlib/Measurements/Three-Phase V-I Measurement  VoltageMeasurement=phase-to-ground  SetLabelV=off  LabelV=Vabc  Vpu=off  VpuLL=off  CurrentMeasurement=yes  SetLabelI=off  LabelI=Iabc  Ipu=off  Pbase=Sbase  Vbase=Vbase*sqrt(3/2)  OutputType=Complex  PhasorSimulation=off  PSBequivalent=0
  Constant2 : Constant  Value=1.05
  Constant4 : Constant  Value=0
  Demux : Demux  Outputs=3
  "Gain 1 " : Gain  Gain=2/3
  Gain1 : Gain  Gain=sqrt(3/2)/WT.Vbase
  Gain2 : Gain  Gain=1/(2*pi*grid.fn)
  Gain9 : Gain  Gain=sqrt(3/2)*WT.Vbase/WT.Sbase
  Goto Tag Visibility1 : GotoTagVisibility  GotoTag=WT_scwt
  I measurement delay WT : TransportDelay  DelayTime=simu.tStep
  Instantaneous Power xyz : pwrsys/Measurement/Instantaneous Power xyz  typeTransf=Amplitude-invariant
      settings: SourceProductName=NTNU Power Systems
  PLL 3-phase abc : pwrsys/PLLs/PLL 3-phase abc  fnom=gsc.fbase  fdev=1/3*gsc.fbase  zeta=0.707  Kp=gsc.pll.Kp  Ki=gsc.pll.Ki  Kd=gsc.pll.Kd  Tr=gsc.pll.Tr  Ts=gsc.fSwitch  wt0=0
      settings: SourceProductName=NTNU Power Systems
  Reactive power x voltage droop Wind Farm : pwrsys/Controllers/Droop controller  Refmax=tan(acos(WT.cosphi))  Refmin=-tan(acos(WT.cosphi))  Ts=-1  Kp=WT.Q.Kp  Kd=WT.Q.Kd  Tr=WT.Q.Tr  flp=WT.Q.flp  DB=WT.Q.DB
      settings: SourceProductName=NTNU Power Systems
  Sqrt1 : Sqrt  SaturateOnIntegerOverflow=on
  Square : Math  Operator=square  SaturateOnIntegerOverflow=on
  Sum of Elements : Sum  Inputs=+
  Sum1 : Sum  Inputs=+-
  Terminator{,1..4} (5 alike) : Terminator
  To Workspace : ToWorkspace  VariableName=WTLog  SaveFormat=Timeseries  SampleTime=-1
      settings: Decimation=20
  V measurement delay WT : TransportDelay  DelayTime=simu.tStep
  Vac lag filter : TransferFcn  Numerator=[0.001 1]  Denominator=[0.01 1]
  WT Grid Side Converter : Subsystem
  abc to xyz : pwrsys/Transformations/abc to xyz  typeTransf=Amplitude-invariant
      settings: SourceProductName=NTNU Power Systems
  abc to xyz1 : pwrsys/Transformations/abc to xyz  typeTransf=Amplitude-invariant
      settings: SourceProductName=NTNU Power Systems
  xyz to dqz : pwrsys/Transformations/xyz to dqz  SystemSampleTime=-1
      settings: SourceProductName=NTNU Power Systems
  xyz to dqz1 : pwrsys/Transformations/xyz to dqz  SystemSampleTime=-1
      settings: SourceProductName=NTNU Power Systems
  A : PMIOPort  Side=Right
  B : PMIOPort  Port=2  Side=Right
  C : PMIOPort  Port=3  Side=Right
  m : Outport
  tag scope: WT_scwt=scoped
  wires:
  I measurement delay WT/1 -> [WT_Iabc]  "Iac"
  Active power x frequency droop Wind Farm/1 -> WT Grid Side Converter/2(Id Ref)  "WT_Idcref"
  Enable/1 -> WT Grid Side Converter/1(Enable)
  V measurement delay WT/1 -> [WT_Vabc]  "Vac"
  Bus 1/1 -> V measurement delay WT/1
  Sum1/1 -> Reactive power x voltage droop Wind Farm/1
  Qsp/1 -> Reactive power x voltage droop Wind Farm/2
  Bus 1/2 -> I measurement delay WT/1
  Vac lag filter/1 -> Active power x frequency droop Wind Farm/3, Reactive power x voltage droop Wind Farm/3
  Reactive power x voltage droop Wind Farm/1 -> WT Grid Side Converter/3(Iq Ref)  "WT_Iqref"
  Psp/1 -> [WT_Pm_pu], Active power x frequency droop Wind Farm/2
  Constant4/1 -> Active power x frequency droop Wind Farm/1
  [WT_Vavg_pu] -> Sum1/2
  Constant2/1 -> Vac lag filter/1, Sum1/1
  Sqrt1/1 -> [WT_Vavg_pu]
  Gain9/1 -> [WT_Iabc_pu], abc to xyz/1  "Iabc_pu"
  xyz to dqz/1 -> [WT_Idq0_pu]  "Idq0_pu"
  Gain1/1 -> Square/1, PLL 3-phase abc/1, [WT_Vabc_pu], abc to xyz1/1  "Vabc_pu"
  PLL 3-phase abc/3 -> [WT_scwt], xyz to dqz/2, xyz to dqz1/2  "scwt"
  Gain2/1 -> [WT_we_pu]  "w"
  PLL 3-phase abc/1 -> Gain2/1
  xyz to dqz1/1 -> [WT_Vdq0_pu]  "Vdq0_pu"
  [WT_Iabc] -> Gain9/1
  [WT_Vabc] -> Gain1/1
  Instantaneous Power xyz/1 -> [WT_Pac_pu]  "Pac_pu"
  Demux/3 -> [WT_Qac_pu]  "Qac_pu"
  Square/1 -> Sum of Elements/1
  Sum of Elements/1 -> "Gain 1 "/1
  "Gain 1 "/1 -> Sqrt1/1
  abc to xyz/1 -> xyz to dqz/1, Instantaneous Power xyz/2  "Ixyz_pu"
  abc to xyz1/1 -> xyz to dqz1/1, Instantaneous Power xyz/1  "Vxyz_pu"
  PLL 3-phase abc/2 -> Terminator/1  "wt"
  Instantaneous Power xyz/2 -> Terminator1/1
  Instantaneous Power xyz/4 -> Terminator2/1
  Instantaneous Power xyz/3 -> Demux/1
  Demux/1 -> Terminator3/1
  Demux/2 -> Terminator4/1
  [WT_Vavg_pu] -> Bus Creator/4  "Vavg"
  [WT_Vdq0_pu] -> Bus Creator/6  "Vdq0"
  [WT_Qac_pu] -> Bus Creator/2  "Q"
  [WT_Idq0_pu] -> Bus Creator/5  "Idq0"
  Bus Creator/1 -> To Workspace/1, m/1  "WT"
  [WT_we_pu] -> Bus Creator/3  "w"
  [WT_Pm_pu] -> Bus Creator/7  "Pm"
  [WT_Pac_pu] -> Bus Creator/1  "Pel"
  [WT_scwt] -> Bus Creator/8  "scwt"
  connections:
  B/RConn1 -- Bus 1/LConn2
  Bus 1/RConn3 -- WT Grid Side Converter/RConn3
  Bus 1/RConn1 -- WT Grid Side Converter/RConn1
  C/RConn1 -- Bus 1/LConn3
  Bus 1/RConn2 -- WT Grid Side Converter/RConn2
  A/RConn1 -- Bus 1/LConn1

== system energy_storage/Energy Storage System/ES1 Battery ==
  Enable : Inport
  Idc Ref : Inport  Port=2
  Controlled Current Source1 : powerlib/Electrical Sources/Controlled Current Source  Initialize=on  Source_Type=DC  Amplitude=0  Phase=0  Frequency=50  Measurements=None
  Enable ES : Product  Inputs=**
  Gain1 : Gain  Gain=es1.Prated/gsc.Sbase
  PWM delay : TransportDelay  DelayTime=simu.tStep
  DC+ : PMIOPort  Side=Right
  DC- : PMIOPort  Port=2  Side=Right
  wires:
  PWM delay/1 -> Controlled Current Source1/1
  Gain1/1 -> Enable ES/2  "ES_Idcref_pu"
  Enable ES/1 -> PWM delay/1  "ES_Idcref_pu"
  Idc Ref/1 -> Gain1/1
  Enable/1 -> Enable ES/1
  connections:
  DC+/RConn1 -- Controlled Current Source1/RConn1
  Controlled Current Source1/LConn1 -- DC-/RConn1

== system energy_storage/Energy Storage System/ES2 Fuel Cell and Electrolyzer ==
  Enable : Inport
  Idc Ref : Inport  Port=2
  Controlled Current Source1 : powerlib/Electrical Sources/Controlled Current Source  Initialize=on  Source_Type=DC  Amplitude=0  Phase=0  Frequency=50  Measurements=None
  Enable ES : Product  Inputs=**
  Gain1 : Gain  Gain=es2.Pely/gsc.Sbase
  PWM delay : TransportDelay  DelayTime=simu.tStep
  DC+ : PMIOPort  Side=Right
  DC- : PMIOPort  Port=2  Side=Right
  wires:
  PWM delay/1 -> Controlled Current Source1/1
  Gain1/1 -> Enable ES/2  "ES_Idcref_pu"
  Enable ES/1 -> PWM delay/1  "ES_Idcref_pu"
  Idc Ref/1 -> Gain1/1
  Enable/1 -> Enable ES/1
  connections:
  Controlled Current Source1/LConn1 -- DC-/RConn1
  Controlled Current Source1/RConn1 -- DC+/RConn1

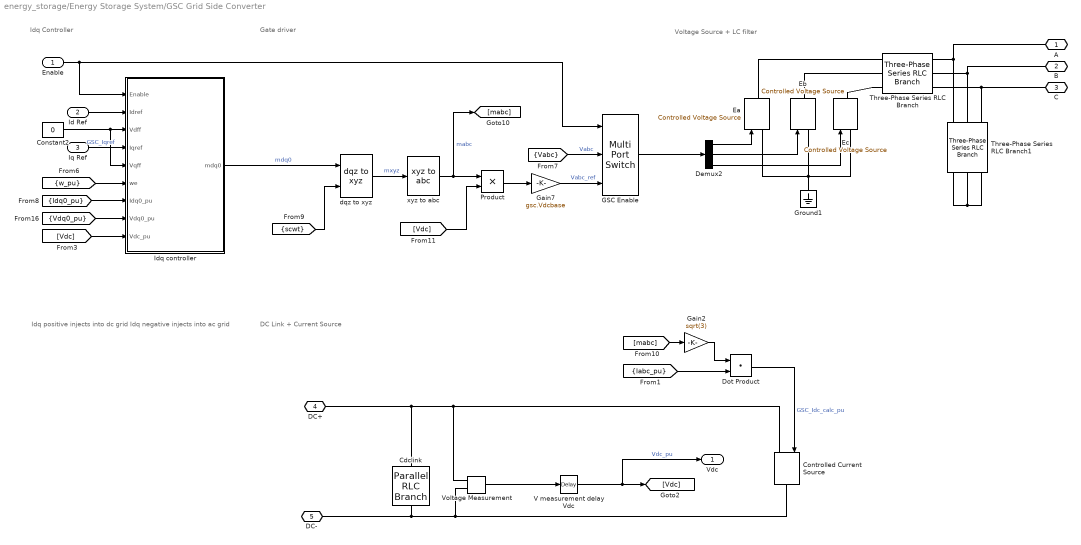
== system energy_storage/Energy Storage System/GSC Grid Side Converter ==
  note: Idq Controller
  note: Gate driver
  note: Voltage Source + LC filter
  note: DC Link + Current Source
  note: Idq positive injects into dc grid
      | Idq negative injects into ac grid
  Enable : Inport
  Id Ref : Inport  Port=2
  Iq Ref : Inport  Port=3
  Cdclink : powerlib/Elements/Parallel RLC Branch  LConnTagsString=a  RConnTagsString=__new0  BranchType=RC  Resistance=1e6  Inductance=0  SetiL0=off  InitialCurrent=0  Capacitance=gsc.filterpu.Cdc  Setx0=on  InitialVoltage=1  Measurements=None
  Constant2 : Constant  Value=0
  Controlled Current Source : powerlib/Electrical Sources/Controlled Current Source  Initialize=on  Source_Type=DC  Amplitude=0  Phase=0  Frequency=0  Measurements=None
  Demux2 : Demux  Outputs=3
  Dot Product : DotProduct  InputSameDT=on  OutDataTypeStr=Inherit: Inherit via internal rule
  Ea : powerlib/Electrical Sources/Controlled Voltage Source  Initialize=on  Source_Type=AC  Amplitude=gsc.Vbase  Phase=0  Frequency=gsc.fbase  Measurements=None
  Eb : powerlib/Electrical Sources/Controlled Voltage Source  Initialize=on  Source_Type=AC  Amplitude=gsc.Vbase  Phase=-120  Frequency=gsc.fbase  Measurements=None
  Ec : powerlib/Electrical Sources/Controlled Voltage Source  Initialize=on  Source_Type=AC  Amplitude=gsc.Vbase  Phase=120  Frequency=gsc.fbase  Measurements=None
  GSC Enable : MultiPortSwitch  DataPortOrder=Zero-based contiguous  Inputs=2  zeroidx=on
  Gain2 : Gain  Gain=sqrt(3)
  Gain7 : Gain  Gain=gsc.Vdcbase
  Ground1 : powerlib/Elements/Ground  LConnTagsString=a
  Idq controller : Subsystem  mask{Imax=1, mmax=gsc.mmax, K=gsc.ctrl.kvsc, Lf=gsc.filterpu.Lac, Rf=gsc.filterpu.Rac, fLC=gsc.ctrl.ffilt, Ts=1/gsc.fSwitch, kp=gsc.ctrl.kp, ki=gsc.ctrl.ki, Kff=1}
      mask prompts: Imax "Maximum AC current"; mmax "Maximum modulation index (PWM gain)"; K "Converter gain (Vdcbase/Vbase)"; Lf "AC filter - L value"; Rf "AC filter - R value"; fLC "AC filter cut-off frequency"; Ts "Sampling time"; Kff "Kff (1 = enable voltage feed-forward)"
      mask DialogControl Container4 Prompt: Controller gains
  Product : Product
  Three-Phase Series RLC Branch : powerlib/Elements/Three-Phase Series RLC Branch  LConnTagsString=A|B|C  RConnTagsString=A|B|C  BranchType=RL  Resistance=gsc.filter.Rac  Inductance=gsc.filter.Lac  Capacitance=1e-6  Measurements=None
  Three-Phase Series RLC Branch1 : powerlib/Elements/Three-Phase Series RLC Branch  LConnTagsString=A|B|C  RConnTagsString=A|B|C  BranchType=RC  Resistance=gsc.filter.Rlc  Inductance=vsc.filter.Lac  Capacitance=gsc.filter.Clc  Measurements=None
  V measurement delay Vdc : TransportDelay  DelayTime=1/gsc.fSwitch
  Voltage Measurement : powerlib/Measurements/Voltage Measurement  PhasorSimulation=off  OutputType=Magnitude  PSBequivalent=0
  dqz to xyz : pwrsys/Transformations/dqz to xyz  SystemSampleTime=-1
      settings: SourceProductName=NTNU Power Systems
  xyz to abc : pwrsys/Transformations/xyz to abc  typeTransf=Amplitude-invariant
      settings: SourceProductName=NTNU Power Systems
  A : PMIOPort  Side=Right
  B : PMIOPort  Port=2  Side=Right
  C : PMIOPort  Port=3  Side=Right
  DC+ : PMIOPort  Port=4  Side=Left
  DC- : PMIOPort  Port=5  Side=Left
  Vdc : Outport
  wires:
  Demux2/2 -> Eb/1
  Demux2/1 -> Ea/1
  Demux2/3 -> Ec/1
  GSC Enable/1 -> Demux2/1
  Idq controller/1(mdq0) -> dqz to xyz/1  "mdq0"
  [Idq0_pu] -> Idq controller/7(Idq0_pu)
  [w_pu] -> Idq controller/6(we)
  [Vdq0_pu] -> Idq controller/8(Vdq0_pu)
  [Vabc] -> GSC Enable/2  "Vabc"
  [scwt] -> dqz to xyz/2
  xyz to abc/1 -> [mabc], Product/1  "mabc"
  Gain7/1 -> GSC Enable/3  "Vabc_ref"
  Constant2/1 -> Idq controller/3(Vdff), Idq controller/5(Vqff)
  dqz to xyz/1 -> xyz to abc/1  "mxyz"
  Iq Ref/1 -> Idq controller/4(Iqref)  "GSC_Iqref"
  Voltage Measurement/1 -> V measurement delay Vdc/1
  Product/1 -> Gain7/1
  Dot Product/1 -> Controlled Current Source/1  "GSC_Idc_calc_pu"
  V measurement delay Vdc/1 -> Vdc/1, [Vdc]  "Vdc_pu"
  [Iabc_pu] -> Dot Product/2
  Gain2/1 -> Dot Product/1
  [Vdc] -> Idq controller/9(Vdc_pu)
  Enable/1 -> Idq controller/1(Enable), GSC Enable/1
  [Vdc] -> Product/2
  [mabc] -> Gain2/1
  Id Ref/1 -> Idq controller/2(Idref)
  connections:
  Three-Phase Series RLC Branch/RConn1 -- Ea/RConn1
  Three-Phase Series RLC Branch/RConn2 -- Eb/RConn1
  Three-Phase Series RLC Branch/RConn3 -- Ec/RConn1
  Three-Phase Series RLC Branch/LConn1 -- A/RConn1 -- Three-Phase Series RLC Branch1/LConn1
  Three-Phase Series RLC Branch1/LConn2 -- Three-Phase Series RLC Branch/LConn2 -- B/RConn1
  Three-Phase Series RLC Branch1/LConn3 -- Three-Phase Series RLC Branch/LConn3 -- C/RConn1
  Ea/LConn1 -- Eb/LConn1 -- Ground1/LConn1 -- Ec/LConn1
  Three-Phase Series RLC Branch1/RConn3 -- Three-Phase Series RLC Branch1/RConn2 -- Three-Phase Series RLC Branch1/RConn1
  Cdclink/RConn1 -- DC-/RConn1 -- Voltage Measurement/LConn2 -- Controlled Current Source/RConn1
  Voltage Measurement/LConn1 -- Controlled Current Source/LConn1 -- DC+/RConn1 -- Cdclink/LConn1

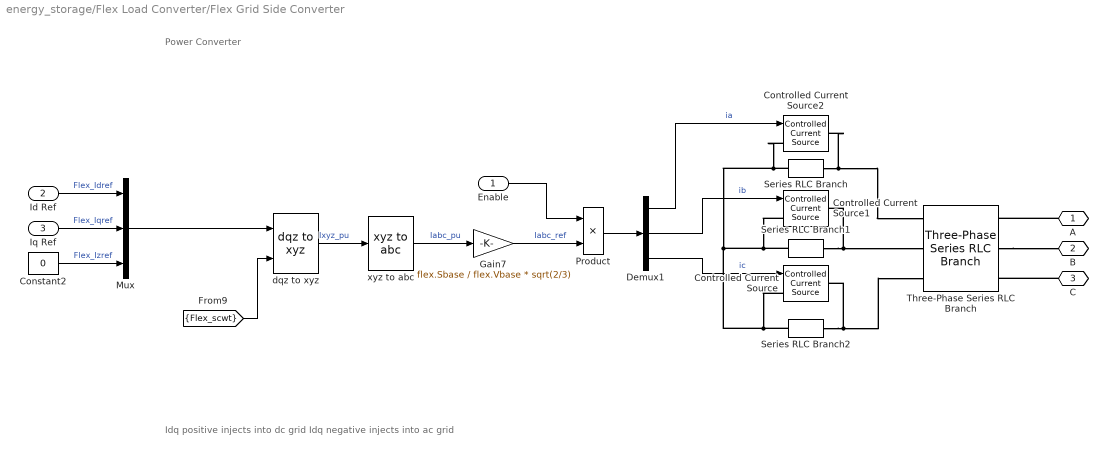
== system energy_storage/Flex Load Converter/Flex Grid Side Converter ==
  note: Power Converter
  note: Idq positive injects into dc grid
      | Idq negative injects into ac grid
  Enable : Inport
  Id Ref : Inport  Port=2
  Iq Ref : Inport  Port=3
  Constant2 : Constant  Value=0
  Controlled Current Source : powerlib/Electrical Sources/Controlled Current Source  Initialize=off  Source_Type=AC  Amplitude=0  Phase=0  Frequency=grid.fn  Measurements=None
  Controlled Current Source1 : powerlib/Electrical Sources/Controlled Current Source  Initialize=off  Source_Type=AC  Amplitude=0  Phase=0  Frequency=grid.fn  Measurements=None
  Controlled Current Source2 : powerlib/Electrical Sources/Controlled Current Source  Initialize=off  Source_Type=AC  Amplitude=0  Phase=0  Frequency=grid.fn  Measurements=None
  Demux1 : Demux  Outputs=3
  Gain7 : Gain  Gain=flex.Sbase / flex.Vbase * sqrt(2/3)
  Mux : Mux  Inputs=3
  Product : Product
  Series RLC Branch : powerlib/Elements/Series RLC Branch  LConnTagsString=__new0  RConnTagsString=__new0  BranchType=RC  Resistance=1e3  Inductance=1e-3  SetiL0=off  InitialCurrent=0  Capacitance=1e3  Setx0=off  InitialVoltage=0  Measurements=None
  Series RLC Branch1 : powerlib/Elements/Series RLC Branch  LConnTagsString=__new0  RConnTagsString=__new0  BranchType=RC  Resistance=1e3  Inductance=1e-3  SetiL0=off  InitialCurrent=0  Capacitance=1e3  Setx0=off  InitialVoltage=0  Measurements=None
  Series RLC Branch2 : powerlib/Elements/Series RLC Branch  LConnTagsString=__new0  RConnTagsString=__new0  BranchType=RC  Resistance=1e3  Inductance=1e-3  SetiL0=off  InitialCurrent=0  Capacitance=1e3  Setx0=off  InitialVoltage=0  Measurements=None
  Three-Phase Series RLC Branch : powerlib/Elements/Three-Phase Series RLC Branch  LConnTagsString=A|B|C  RConnTagsString=A|B|C  BranchType=RL  Resistance=flex.filter.Rac  Inductance=flex.filter.Lac  Capacitance=1e-6  Measurements=None
  dqz to xyz : pwrsys/Transformations/dqz to xyz  SystemSampleTime=-1
      settings: SourceProductName=NTNU Power Systems
  xyz to abc : pwrsys/Transformations/xyz to abc  typeTransf=Amplitude-invariant
      settings: SourceProductName=NTNU Power Systems
  A : PMIOPort  Side=Right
  B : PMIOPort  Port=2  Side=Right
  C : PMIOPort  Port=3  Side=Right
  wires:
  [Flex_scwt] -> dqz to xyz/2
  xyz to abc/1 -> Gain7/1  "Iabc_pu"
  Gain7/1 -> Product/2  "Iabc_ref"
  dqz to xyz/1 -> xyz to abc/1  "Ixyz_pu"
  Enable/1 -> Product/1
  Id Ref/1 -> Mux/1  "Flex_Idref"
  Iq Ref/1 -> Mux/2  "Flex_Iqref"
  Constant2/1 -> Mux/3  "Flex_Izref"
  Mux/1 -> dqz to xyz/1
  Demux1/1 -> Controlled Current Source2/1  "ia"
  Demux1/2 -> Controlled Current Source1/1  "ib"
  Product/1 -> Demux1/1
  Demux1/3 -> Controlled Current Source/1  "ic"
  connections:
  Controlled Current Source/RConn1 -- Three-Phase Series RLC Branch/RConn3 -- Series RLC Branch2/LConn1
  Controlled Current Source2/RConn1 -- Three-Phase Series RLC Branch/RConn1 -- Series RLC Branch/LConn1
  Controlled Current Source1/RConn1 -- Three-Phase Series RLC Branch/RConn2 -- Series RLC Branch1/LConn1
  Series RLC Branch1/RConn1 -- Controlled Current Source1/LConn1 -- Controlled Current Source/LConn1 -- Series RLC Branch2/RConn1 -- Controlled Current Source2/LConn1 -- Series RLC Branch/RConn1
  A/RConn1 -- Three-Phase Series RLC Branch/LConn1
  C/RConn1 -- Three-Phase Series RLC Branch/LConn3
  Three-Phase Series RLC Branch/LConn2 -- B/RConn1

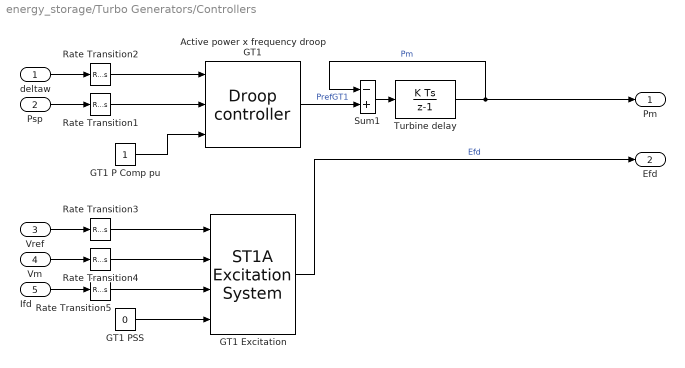
== system energy_storage/Turbo Generators/Controllers ==
  deltaw : Inport
  Psp : Inport  Port=2
  Vref : Inport  Port=3
  Vm : Inport  Port=4
  Ifd : Inport  Port=5
  Active power x frequency droop GT1 : pwrsys/Controllers/Droop controller  Refmax=SMcosphi  Refmin=0  Ts=1/(20*grid.fn)  Kp=GovKp  Kd=GovKd  Tr=GovTr  flp=GovFlp  DB=GovDB
      settings: SourceProductName=NTNU Power Systems
  GT1 Excitation : sps_avr/ST1A Excitation System  Tr=ExcTr  KaTa=[ExcKa 1/(6*SMfn)]  VIminmax=[-0.2 0.2]  VAminmax=[ExcVRMin ExcVRMax]  VRminmax=[ExcVRMin ExcVRMax]  KfTf=[ExcKf ExcTf]  TbTc=[ExcTb ExcTc ExcTb1 ExcTc1]  KLR=0  ILR=999  Kc=0  v0=[1,sqrt(3/2)*1.27233]  TsBlock=1/(20*grid.fn)
      settings: SourceProductName=Simscape Power Systems  SourceProductBaseCode=PS
  GT1 P Comp pu : Constant  SampleTime=-1
  GT1 PSS : Constant  Value=0  SampleTime=-1
  Rate Transition{1..5} (5 alike) : RateTransition
  Sum1 : Sum  Inputs=-+
  Turbine delay : DiscreteIntegrator  gainval=1/TurbT  InitialCondition=gt1.P.Ref  SampleTime=-1  LimitOutput=on  UpperSaturationLimit=SMcosphi  LowerSaturationLimit=0  ICPrevOutput=DiscIntNeverNeededParam  ICPrevScaledInput=DiscIntNeverNeededParam
  Pm : Outport
  Efd : Outport  Port=2
  wires:
  Vref/1 -> Rate Transition3/1
  Vm/1 -> Rate Transition4/1
  Active power x frequency droop GT1/1 -> Sum1/2  "PrefGT1"
  GT1 PSS/1 -> GT1 Excitation/4
  Turbine delay/1 -> Pm/1, Sum1/1  "Pm"
  GT1 Excitation/1 -> Efd/1  "Efd"
  GT1 P Comp pu/1 -> Active power x frequency droop GT1/3
  Ifd/1 -> Rate Transition5/1
  Sum1/1 -> Turbine delay/1
  Psp/1 -> Rate Transition1/1
  deltaw/1 -> Rate Transition2/1
  Rate Transition2/1 -> Active power x frequency droop GT1/1
  Rate Transition1/1 -> Active power x frequency droop GT1/2
  Rate Transition3/1 -> GT1 Excitation/1
  Rate Transition4/1 -> GT1 Excitation/2
  Rate Transition5/1 -> GT1 Excitation/3
